simulink model "sibBuilderBlock_TestGen2"  (R2017b)
settings: Solver=FixedStepDiscrete  StartTime=0.0  StopTime=10.0  RelTol=1e-3
undefined symbols (not defined in the file): sigbuilder_block
settings Model: Creator=ktrinh  LastModifiedBy=ktrinh
settings DebuggingCC: ParameterOverflowMsg=none

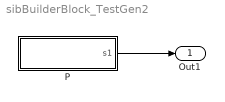
== system sibBuilderBlock_TestGen2 ==
  P : Subsystem  Tag=STV Subsys  LoadFcn=sigbuilder_block('load',[50 52 520 400 ]);  StartFcn=sigbuilder_block('start');  StopFcn=sigbuilder_block('stop');  ClipboardFcn=sigbuilder_block('clipboard');  mask(Sigbuilder block){tuvar=[0:10]}
      mask init:
      | if ~strcmp(get_param(bdroot(gcb),'SimulationStatus'),'stopped'),tuvar = sigbuilder_block('maskInit'); end
      settings: CopyFcn=sigbuilder_block('copy');  DeleteFcn=sigbuilder_block('delete');  ModelCloseFcn=sigbuilder_block('modelClose');  PreSaveFcn=sigbuilder_block('preSave');  PauseFcn=sigbuilder_block('pause');  ContinueFcn=sigbuilder_block('continue');  NameChangeFcn=sigbuilder_block('namechange');  OpenFcn=sigbuilder_block('open');  CloseFcn=sigbuilder_block('close');
      mask Display: plot(0, 0, 100, 100,[2, 2, 32, 32, 2], [68, 8, 8, 68, 68],[32, 2], [38, 38], [32, 19, 2],[53, 60, 44], [32, 17, 17, 2],[16, 16, 31, 31]);txt = getActiveGroup(gcbh);text(2, 100, txt,'verticalAlignment', 'top');
  Out1 : Outport
  wires:
  P/1(s1) -> Out1/1

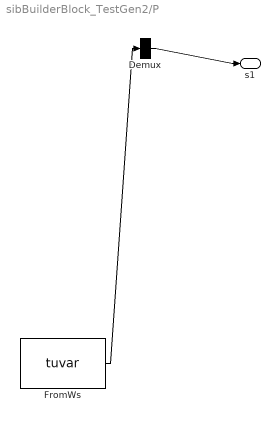
== system sibBuilderBlock_TestGen2/P ==
  Demux : Demux  Tag=STV Demux  Outputs=1
  FromWs : FromWorkspace  Tag=STV FromWs  VariableName=tuvar  SampleTime=0
      SigBuilderData=|
      | dataSet.timeRange = [0 9.8]
      | dataSet.name = 'group1'
      | sbobj.Name = 'Signal Builder'
      | sbobj.Groups.Name = 'group1'
      | sbobj.Groups.Signals.Name = 's1'
      | sbobj.Groups.Signals.XData = [0 0.2 0.4 0.6 0.8 1 1.2 1.4 1.6 1.8 2 2.2 2.4 2.6 2.8 3 3.2 3.4 3.6 3.8 4 4.2 4.4 4.6 4.8 5 5.2 5.4 5.6 5.8 6 6.2 6.4 6.6 6.8 7 7.2 7.4 7.6 7.8 8 8.2 8.4 8.6 8.8 9 9.2 9.4 9.6 9.8]
      | sbobj.Groups.Signals.YData = [0 0.198669330795 0.389418342309 0.564642473395 0.7173560909 0.841470984808 0.932039085967 0.985449729988 0.999573603042 0.973847630878 0.909297426826 0.80849640382 0.675463180551 0.515501371821 0.334988150156 0.14112000806 -0.0583741434276 -0.255541102027 -0.442520443295 -0.611857890943 -0.756802495308 -0.871575772414 -0.95160207389 -0.993691003633 -0.996164608836 -0.958924274663 -0.88345465572 -0.772764487556 -0.631266637872 -0.464602179414 -0.279415498199 -0.0830894028175 0.11654920485 0.311541363513 0.494113351139 0.656986598719 0.793667863849 0.898708095812 0.967919672031 0.998543345375 0.989358246623 0.94073055668 0.854598908088 0.734397097874 0.584917192892 0.412118485242 0.2228899141 0.0247754254534 -0.174326781223 -0.366479129252]
      | sbobj.Groups.TimeRange = [0 9.8]
  s1 : Outport  Tag=STV Outport
  wires:
  FromWs/1 -> Demux/1
  Demux/1 -> s1/1
